simulink model "AUAV3_WITH_SLUGS_SENSOR_AND_CONTROLLER"  (Simulink 8.5)
settings: Solver=FixedStepDiscrete  StartTime=0.0  StopTime=10.0  FixedStep=T  RelTol=1e-3
PreLoadFcn:
  | T = 0.0025;
  | MavlinkBus;
  | 
  | % Baro Altitude Computation
  | % =========================
  | basePressure = 98192.64;
  | baseTemp = 288.215;
  | lapseRate = -0.00198122;
  | baseHeight = 0;
  | 
  | mcuInit
values from neighbouring files (symbols this model uses):
  apSampleTime = 0.01    [mcuInit.m]
  latlong_WP = 1    [mcuInit.m]
  mavlink_gps_raw_int_t = Simulink.Bus    [MavlinkBus.m]    (also in MavlinkBusMarcello.m)
  mavlink_raw_imu_t = Simulink.Bus    [MavlinkBus.m]    (also in MavlinkBusMarcello.m)
  mavlink_scaled_pressure_t = Simulink.Bus    [MavlinkBus.m]    (also in MavlinkBusMarcello.m)
  mavlink_sys_status_t = Simulink.Bus    [MavlinkBus.m]    (also in MavlinkBusMarcello.m)
  Xpoints = [0 0]    [mcuInit.m]
  Ypoints = [0 0]    [mcuInit.m]
  Zpoints = [0 0]    [mcuInit.m]
undefined symbols (not defined in the file or in its folder): A0, A14, A15, A2, A3, A5, A6, accBiasRateLimit, altLatLon, B0, bankCommandLimit, barAdjust, baroCutoff, baroCutTemp, C3, cubeAccelGain16405, cubeGyroGain16405, cubeMagGain16405, D0, D11, D13, D8, daLimit, data, daTrimMax, daTrimMin, deLimit, deTrimMax, deTrimMin, drLimit, drTrimMax, drTrimMin, dtLimit, dtTrimMax, dtTrimMin, F2, F3, G0, G15, gaind, GS_location, gyroBiasRateLimit, IC1max, IPStar, ISA_g, maxAcc, MaxDwnPthStar, maxDynPressure, maxEta, OC1max, P112, P127, P16, P21, P30, P31, P51, P64, P72, P75 ... (+39)
undefined symbols (not defined in the file): baroOffset, baroScale, barTGain1, barTGain2, barTMean1, barTMean2, bda, bde, bdr, bdt, bICda, bICde, bICdr, bICdt, derivativesConstant, lowRateSensorCutoff, mainSensorCutoff, mda, mde, mdr, mdt, mICda, mICde, mICdr, mICdt, pitotOffset, pitotScale, pitTGain1, pitTGain2, pitTMean1, pitTMean2, powerOffset, powerScale, pressureSensorCutoff, tempOffset, tempScale, vzCutoff, xCutoff, yCutoff
libraries: MCHP_Blockset x147, simulink x78, SLUGS_Library x31, aerolibconvert2 x6, aerolibutil x4, aerolibtransform2 x3, dspmtrx3 x2, aerolibobsolete x2
(part 2 of 12)

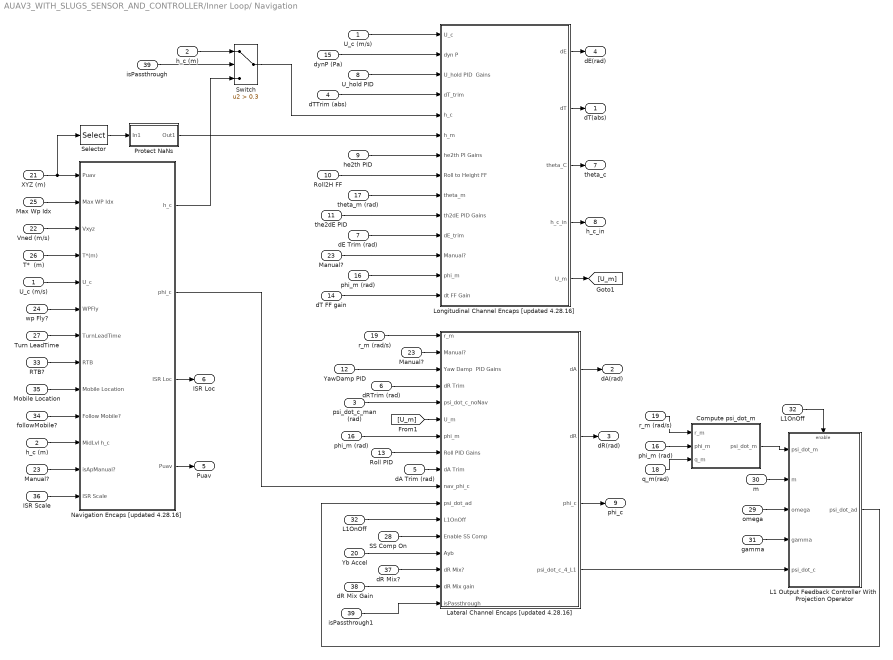
== system AUAV3_WITH_SLUGS_SENSOR_AND_CONTROLLER/Inner Loop/ Navigation ==
  U_c (m/s) : Inport
  h_c (m) : Inport  Port=2
  psi_dot_c_man (rad) : Inport  Port=3
  dTTrim (abs) : Inport  Port=4
  dA Trim (rad) : Inport  Port=5
  dRTrim (rad) : Inport  Port=6
  dE Trim (rad) : Inport  Port=7
  U_hold PID : Inport  Port=8
  he2th PID : Inport  Port=9
  Roll2H FF : Inport  Port=10
  the2dE PID : Inport  Port=11
  YawDamp PID : Inport  Port=12
  "Roll PID " : Inport  Port=13
  dT FF gain : Inport  Port=14
  dynP (Pa) : Inport  Port=15
  phi_m (rad) : Inport  Port=16
  theta_m (rad) : Inport  Port=17
  q_m(rad) : Inport  Port=18
  r_m (rad/s) : Inport  Port=19
  Yb Accel : Inport  Port=20
  XYZ (m) : Inport  Port=21
  Vned (m/s) : Inport  Port=22
  Manual? : Inport  Port=23
  wp Fly? : Inport  Port=24
  Max Wp Idx : Inport  Port=25
  T*  (m) : Inport  Port=26
  Turn LeadTime : Inport  Port=27
  SS Comp On : Inport  Port=28
  omega : Inport  Port=29
  m : Inport  Port=30
  gamma : Inport  Port=31
  L1OnOff : Inport  Port=32
  RTB? : Inport  Port=33
  followMobile? : Inport  Port=34
  Mobile Location : Inport  Port=35
  ISR Scale : Inport  Port=36
  dR Mix? : Inport  Port=37
  dR Mix Gain : Inport  Port=38
  isPassthrough : Inport  Port=39
  Compute psi_dot_m : Subsystem
  L1 Output Feedback Controller With  Projection Operator : Subsystem  TreatAsAtomicUnit=on
  "L1OnOff " : InportShadow  Port=32
  Lateral Channel Encaps [updated 4.28.16] : Subsystem  TreatAsAtomicUnit=on
  Longitudinal Channel Encaps [updated 4.28.16] : Subsystem  TreatAsAtomicUnit=on
  "Manual? " : InportShadow  Port=23
  "Manual?  " : InportShadow  Port=23
  Navigation Encaps [updated 4.28.16] : Subsystem  TreatAsAtomicUnit=on
  Protect NaNs : Subsystem
  Selector : Selector  InputPortWidth=3  Indices=[3]
  Switch : Switch  Criteria=u2 > Threshold  Threshold=0.3  OutDataTypeStr=Inherit: Inherit via back propagation  InputSameDT=on
  "U_c (m/s) " : InportShadow
  "h_c (m) " : InportShadow  Port=2
  isPassthrough1 : InportShadow  Port=39
  "phi_m (rad) " : InportShadow  Port=16
  "phi_m (rad)   " : InportShadow  Port=16
  "r_m (rad/s) " : InportShadow  Port=19
  dT(abs) : Outport
  dA(rad) : Outport  Port=2
  dR(rad) : Outport  Port=3
  dE(rad) : Outport  Port=4
  "Puav " : Outport  Port=5
  ISR Loc : Outport  Port=6
  theta_c : Outport  Port=7
  h_c_in : Outport  Port=8
  phi_c : Outport  Port=9
  wires:
  Manual?/1 -> Longitudinal Channel Encaps [updated 4.28.16]/12(Manual?)
  U_c (m/s)/1 -> Longitudinal Channel Encaps [updated 4.28.16]/1(U_c)
  dynP (Pa)/1 -> Longitudinal Channel Encaps [updated 4.28.16]/2(dyn P)
  Longitudinal Channel Encaps [updated 4.28.16]/1(dE) -> dE(rad)/1
  U_hold PID/1 -> Longitudinal Channel Encaps [updated 4.28.16]/3(U_hold PID  Gains)
  dTTrim (abs)/1 -> Longitudinal Channel Encaps [updated 4.28.16]/4(dT_trim)
  Longitudinal Channel Encaps [updated 4.28.16]/2(dT) -> dT(abs)/1
  Selector/1 -> Protect NaNs/1(In1)
  he2th PID/1 -> Longitudinal Channel Encaps [updated 4.28.16]/7(he2th PI Gains)
  theta_m (rad)/1 -> Longitudinal Channel Encaps [updated 4.28.16]/9(theta_m)
  Longitudinal Channel Encaps [updated 4.28.16]/3(theta_C) -> theta_c/1
  the2dE PID/1 -> Longitudinal Channel Encaps [updated 4.28.16]/10(th2dE PID Gains)
  dE Trim (rad)/1 -> Longitudinal Channel Encaps [updated 4.28.16]/11(dE_trim)
  Longitudinal Channel Encaps [updated 4.28.16]/4(h_c_in) -> h_c_in/1
  r_m (rad/s)/1 -> Lateral Channel Encaps [updated 4.28.16]/1(r_m)
  YawDamp PID/1 -> Lateral Channel Encaps [updated 4.28.16]/3(Yaw Damp  PID Gains)
  dRTrim (rad)/1 -> Lateral Channel Encaps [updated 4.28.16]/4(dR Trim)
  Lateral Channel Encaps [updated 4.28.16]/2(dR) -> dR(rad)/1
  psi_dot_c_man (rad)/1 -> Lateral Channel Encaps [updated 4.28.16]/5(psi_dot_c_noNav)
  phi_m (rad)/1 -> Lateral Channel Encaps [updated 4.28.16]/7(phi_m)
  Lateral Channel Encaps [updated 4.28.16]/3(phi_c) -> phi_c/1
  "Roll PID "/1 -> Lateral Channel Encaps [updated 4.28.16]/8(Roll PID Gains)
  dA Trim (rad)/1 -> Lateral Channel Encaps [updated 4.28.16]/9(dA Trim)
  Longitudinal Channel Encaps [updated 4.28.16]/5(U_m) -> [U_m]
  XYZ (m)/1 -> Selector/1, Navigation Encaps [updated 4.28.16]/1(Puav)
  Max Wp Idx/1 -> Navigation Encaps [updated 4.28.16]/2(Max WP Idx)
  Vned (m/s)/1 -> Navigation Encaps [updated 4.28.16]/3(Vxyz)
  Compute psi_dot_m/1(psi_dot_m) -> L1 Output Feedback Controller With  Projection Operator/1(psi_dot_m)
  m/1 -> L1 Output Feedback Controller With  Projection Operator/2(m)
  omega/1 -> L1 Output Feedback Controller With  Projection Operator/3(omega)
  gamma/1 -> L1 Output Feedback Controller With  Projection Operator/4(gamma)
  "r_m (rad/s) "/1 -> Compute psi_dot_m/1(r_m)
  "phi_m (rad) "/1 -> Compute psi_dot_m/2(phi_m)
  q_m(rad)/1 -> Compute psi_dot_m/3(q_m)
  L1OnOff/1 -> L1 Output Feedback Controller With  Projection Operator/Enable
  L1 Output Feedback Controller With  Projection Operator/1(psi_dot_ad) -> Lateral Channel Encaps [updated 4.28.16]/11(psi_dot_ad)
  "L1OnOff "/1 -> Lateral Channel Encaps [updated 4.28.16]/12(L1OnOff)
  "phi_m (rad)   "/1 -> Longitudinal Channel Encaps [updated 4.28.16]/13(phi_m)
  dT FF gain/1 -> Longitudinal Channel Encaps [updated 4.28.16]/14(dt FF Gain)
  Lateral Channel Encaps [updated 4.28.16]/1(dA) -> dA(rad)/1
  SS Comp On/1 -> Lateral Channel Encaps [updated 4.28.16]/13(Enable SS Comp)
  Yb Accel/1 -> Lateral Channel Encaps [updated 4.28.16]/14(Ayb)
  Lateral Channel Encaps [updated 4.28.16]/4(psi_dot_c_4_L1) -> L1 Output Feedback Controller With  Projection Operator/5(psi_dot_c)
  Protect NaNs/1(Out1) -> Longitudinal Channel Encaps [updated 4.28.16]/6(h_m)
  [U_m] -> Lateral Channel Encaps [updated 4.28.16]/6(U_m)
  "Manual?  "/1 -> Lateral Channel Encaps [updated 4.28.16]/2(Manual?)
  Roll2H FF/1 -> Longitudinal Channel Encaps [updated 4.28.16]/8(Roll to Height FF)
  Navigation Encaps [updated 4.28.16]/2(phi_c) -> Lateral Channel Encaps [updated 4.28.16]/10(nav_phi_c)
  T*  (m)/1 -> Navigation Encaps [updated 4.28.16]/4(T*(m))
  "U_c (m/s) "/1 -> Navigation Encaps [updated 4.28.16]/5(U_c)
  wp Fly?/1 -> Navigation Encaps [updated 4.28.16]/6(WPFly)
  Turn LeadTime/1 -> Navigation Encaps [updated 4.28.16]/7(TurnLeadTime)
  RTB?/1 -> Navigation Encaps [updated 4.28.16]/8(RTB)
  Mobile Location/1 -> Navigation Encaps [updated 4.28.16]/9(Mobile Location)
  followMobile?/1 -> Navigation Encaps [updated 4.28.16]/10(Follow Mobile?)
  "h_c (m) "/1 -> Navigation Encaps [updated 4.28.16]/11(MidLvl h_c)
  "Manual? "/1 -> Navigation Encaps [updated 4.28.16]/12(isApManual?)
  Navigation Encaps [updated 4.28.16]/3(ISR Loc) -> ISR Loc/1
  Navigation Encaps [updated 4.28.16]/4("Puav ") -> "Puav "/1
  dR Mix Gain/1 -> Lateral Channel Encaps [updated 4.28.16]/16(dR Mix gain)
  dR Mix?/1 -> Lateral Channel Encaps [updated 4.28.16]/15(dR Mix?)
  ISR Scale/1 -> Navigation Encaps [updated 4.28.16]/13(ISR Scale)
  isPassthrough/1 -> Switch/2
  h_c (m)/1 -> Switch/1
  Switch/1 -> Longitudinal Channel Encaps [updated 4.28.16]/5(h_c)
  Navigation Encaps [updated 4.28.16]/1(h_c) -> Switch/3
  isPassthrough1/1 -> Lateral Channel Encaps [updated 4.28.16]/17(isPassthrough)

== system AUAV3_WITH_SLUGS_SENSOR_AND_CONTROLLER/MavlinkTX ==
  COMP_ID : Constant  OutDataTypeStr=uint8
  Get Raw IMU : DataStoreRead  DataStoreName=mlRawIMU  DataStoreElements=mlRawIMU
  Get RawGpsInt : DataStoreRead  DataStoreName=mlGpsData
  Get mlAirData : DataStoreRead  DataStoreName=mlAirData  DataStoreElements=mlAirData
  Get mlSysStatus : DataStoreRead  DialogController=Simulink.DDGSource  DataStoreName=mlSysStatus  DataStoreElements=mlSysStatus
  Get time : DataStoreRead  DataStoreName=time_since_boot_usec  DataStoreElements=time_since_boot_usec
  Get time1 : DataStoreRead  DataStoreName=time_since_boot_usec  DataStoreElements=time_since_boot_usec
  Get time2 : DataStoreRead  DataStoreName=time_since_boot_usec  DataStoreElements=time_since_boot_usec
  PackGpsRawInt : MCHP_Blockset/User Functions/C Function Call  ParseFilesChkbx=off  ListFunctions1=Custom Function  Function1=uint16_t PackGpsRawInt(uint8_t system_id, uint8_t component_id, mavlink_gps_raw_int_t mlRawGpsDataInt ,uint32_t time_usec)  AddHeaderDeclaration=on  Function1Type=when block is updated (default)  Fct1BlockIn="system_id  , component_id  , mlRawGpsDataInt  , time_usec"  FctReturnBlockOut=on  DataCollected=0  ORDERING=None  SampleTime=0.2  MCHP_MASTERLINK=|  PinDigitalInput=[]  PinDigitalOutput=[]  PinAnalogInput=[]
      | AUAV3_WITH_SLUGS_SENSOR_AND_CONTROLLER/Microchip Master
      | AUAV V3 Board
      | Busy Flag on D2 (RA6)
  PackHeartBeat : MCHP_Blockset/User Functions/C Function Call  ParseFilesChkbx=off  ListFunctions1=Custom Function  Function1=uint16_t PackHeartBeat(uint8_t system_id, uint8_t component_id)  AddHeaderDeclaration=on  Function1Type=when block is updated (default)  Fct1BlockIn="system_id  , component_id"  FctReturnBlockOut=on  DataCollected=0  ORDERING=None  SampleTime=0.5  MCHP_MASTERLINK=|  PinDigitalInput=[]  PinDigitalOutput=[]  PinAnalogInput=[]
      | AUAV3_WITH_SLUGS_SENSOR_AND_CONTROLLER/Microchip Master
      | AUAV V3 Board
      | Busy Flag on D2 (RA6)
  PackRawIMU : MCHP_Blockset/User Functions/C Function Call  ParseFilesChkbx=off  ListFunctions1=Custom Function  Function1=uint16_t PackRawIMU(uint8_t system_id, uint8_t component_id, mavlink_raw_imu_t mlRawIMUData ,uint32_t time_usec)  AddHeaderDeclaration=on  Function1Type=when block is updated (default)  Fct1BlockIn="system_id  , component_id  , mlRawIMUData  , time_usec"  FctReturnBlockOut=on  DataCollected=0  ORDERING=None  SampleTime=0.02  MCHP_MASTERLINK=|  PinDigitalInput=[]  PinDigitalOutput=[]  PinAnalogInput=[]
      | AUAV3_WITH_SLUGS_SENSOR_AND_CONTROLLER/Microchip Master
      | AUAV V3 Board
      | Busy Flag on D2 (RA6)
  PackScaledPressure : MCHP_Blockset/User Functions/C Function Call  ParseFilesChkbx=off  ListFunctions1=Custom Function  Function1=uint16_t PackScaledPressure(uint8_t system_id, uint8_t component_id, mavlink_scaled_pressure_t mlAirData ,uint32_t time_usec)  AddHeaderDeclaration=on  Function1Type=when block is updated (default)  Fct1BlockIn="system_id  , component_id  , mlAirData  , time_usec"  FctReturnBlockOut=on  DataCollected=0  ORDERING=None  SampleTime=[0.2 0.02]  MCHP_MASTERLINK=|  PinDigitalInput=[]  PinDigitalOutput=[]  PinAnalogInput=[]
      | AUAV3_WITH_SLUGS_SENSOR_AND_CONTROLLER/Microchip Master
      | AUAV V3 Board
      | Busy Flag on D2 (RA6)
  PackSysStatus : MCHP_Blockset/User Functions/C Function Call  ParseFilesChkbx=off  ListFunctions1=Custom Function  Function1=uint16_t PackSysStatus(uint8_t system_id, uint8_t component_id, mavlink_sys_status_t mlSysStatus)  AddHeaderDeclaration=on  Function1Type=when block is updated (default)  Fct1BlockIn="system_id  , component_id  , mlSysStatus"  FctReturnBlockOut=on  DataCollected=0  ORDERING=None  SampleTime=[0.2 0.04]  MCHP_MASTERLINK=|  PinDigitalInput=[]  PinDigitalOutput=[]  PinAnalogInput=[]
      | AUAV3_WITH_SLUGS_SENSOR_AND_CONTROLLER/Microchip Master
      | AUAV V3 Board
      | Busy Flag on D2 (RA6)
  ParamInterfaceResponse : MCHP_Blockset/User Functions/C Function Call  ParseFilesChkbx=off  ListFunctions1=Custom Function  Function1=uint16_t ParameterInterfaceResponse(uint8_t system_id, uint8_t component_id)  AddHeaderDeclaration=on  Function1Type=when block is updated (default)  Fct1BlockIn="system_id  , component_id"  FctReturnBlockOut=on  DataCollected=0  ORDERING=None  SampleTime=[0.2 0.06]  MCHP_MASTERLINK=|  PinDigitalInput=[]  PinDigitalOutput=[]  PinAnalogInput=[]
      | AUAV3_WITH_SLUGS_SENSOR_AND_CONTROLLER/Microchip Master
      | AUAV V3 Board
      | Busy Flag on D2 (RA6)
  ParamInterfaceResponse1 : MCHP_Blockset/User Functions/C Function Call  ParseFilesChkbx=off  ListFunctions1=Custom Function  Function1=uint16_t MissionInterfaceResponse(uint8_t system_id, uint8_t component_id)  AddHeaderDeclaration=on  Function1Type=when block is updated (default)  Fct1BlockIn="system_id  , component_id"  FctReturnBlockOut=on  DataCollected=0  ORDERING=None  SampleTime=[0.2 0.08]  MCHP_MASTERLINK=|  PinDigitalInput=[]  PinDigitalOutput=[]  PinAnalogInput=[]
      | AUAV3_WITH_SLUGS_SENSOR_AND_CONTROLLER/Microchip Master
      | AUAV V3 Board
      | Busy Flag on D2 (RA6)
  SYS_ID : Constant  Value=101  OutDataTypeStr=uint8
  TX_N_Data : MCHP_Blockset/User Functions/C Function Call  ParseFilesChkbx=off  ListFunctions1=Custom Function  Function1=void TxN_Data_OverU1(uint16_t N)  AddHeaderDeclaration=on  Function1Type=when block is updated (default)  Fct1BlockIn=N  FctReturnBlockOut=on  DataCollected=0  ORDERING=None  SampleTime=-1  MCHP_MASTERLINK=|  PinDigitalInput=[]  PinDigitalOutput=[]  PinAnalogInput=[]
      | AUAV3_WITH_SLUGS_SENSOR_AND_CONTROLLER/Microchip Master
      | AUAV V3 Board
      | Busy Flag on D2 (RA6)
  TX_N_Data1 : MCHP_Blockset/User Functions/C Function Call  ParseFilesChkbx=off  ListFunctions1=Custom Function  Function1=void TxN_Data_OverU1(uint16_t N)  AddHeaderDeclaration=on  Function1Type=when block is updated (default)  Fct1BlockIn=N  FctReturnBlockOut=on  DataCollected=0  ORDERING=None  SampleTime=-1  MCHP_MASTERLINK=|  PinDigitalInput=[]  PinDigitalOutput=[]  PinAnalogInput=[]
      | AUAV3_WITH_SLUGS_SENSOR_AND_CONTROLLER/Microchip Master
      | AUAV V3 Board
      | Busy Flag on D2 (RA6)
  TX_N_Data2 : MCHP_Blockset/User Functions/C Function Call  ParseFilesChkbx=off  ListFunctions1=Custom Function  Function1=void TxN_Data_OverU1(uint16_t N)  AddHeaderDeclaration=on  Function1Type=when block is updated (default)  Fct1BlockIn=N  FctReturnBlockOut=on  DataCollected=0  ORDERING=None  SampleTime=-1  MCHP_MASTERLINK=|  PinDigitalInput=[]  PinDigitalOutput=[]  PinAnalogInput=[]
      | AUAV3_WITH_SLUGS_SENSOR_AND_CONTROLLER/Microchip Master
      | AUAV V3 Board
      | Busy Flag on D2 (RA6)
  TX_N_Data3 : MCHP_Blockset/User Functions/C Function Call  ParseFilesChkbx=off  ListFunctions1=Custom Function  Function1=void TxN_Data_OverU1(uint16_t N)  AddHeaderDeclaration=on  Function1Type=when block is updated (default)  Fct1BlockIn=N  FctReturnBlockOut=on  DataCollected=0  ORDERING=None  SampleTime=-1  MCHP_MASTERLINK=|  PinDigitalInput=[]  PinDigitalOutput=[]  PinAnalogInput=[]
      | AUAV3_WITH_SLUGS_SENSOR_AND_CONTROLLER/Microchip Master
      | AUAV V3 Board
      | Busy Flag on D2 (RA6)
  TX_N_Data4 : MCHP_Blockset/User Functions/C Function Call  ParseFilesChkbx=off  ListFunctions1=Custom Function  Function1=void TxN_Data_OverU1(uint16_t N)  AddHeaderDeclaration=on  Function1Type=when block is updated (default)  Fct1BlockIn=N  FctReturnBlockOut=on  DataCollected=0  ORDERING=None  SampleTime=-1  MCHP_MASTERLINK=|  PinDigitalInput=[]  PinDigitalOutput=[]  PinAnalogInput=[]
      | AUAV3_WITH_SLUGS_SENSOR_AND_CONTROLLER/Microchip Master
      | AUAV V3 Board
      | Busy Flag on D2 (RA6)
  TX_N_Data5 : MCHP_Blockset/User Functions/C Function Call  ParseFilesChkbx=off  ListFunctions1=Custom Function  Function1=void TxN_Data_OverU1(uint16_t N)  AddHeaderDeclaration=on  Function1Type=when block is updated (default)  Fct1BlockIn=N  FctReturnBlockOut=on  DataCollected=0  ORDERING=None  SampleTime=-1  MCHP_MASTERLINK=|  PinDigitalInput=[]  PinDigitalOutput=[]  PinAnalogInput=[]
      | AUAV3_WITH_SLUGS_SENSOR_AND_CONTROLLER/Microchip Master
      | AUAV V3 Board
      | Busy Flag on D2 (RA6)
  TX_N_Data6 : MCHP_Blockset/User Functions/C Function Call  ParseFilesChkbx=off  ListFunctions1=Custom Function  Function1=void TxN_Data_OverU1(uint16_t N)  AddHeaderDeclaration=on  Function1Type=when block is updated (default)  Fct1BlockIn=N  FctReturnBlockOut=on  DataCollected=0  ORDERING=None  SampleTime=-1  MCHP_MASTERLINK=|  PinDigitalInput=[]  PinDigitalOutput=[]  PinAnalogInput=[]
      | AUAV3_WITH_SLUGS_SENSOR_AND_CONTROLLER/Microchip Master
      | AUAV V3 Board
      | Busy Flag on D2 (RA6)
  wires:
  Get mlSysStatus/1 -> ?
  PackSysStatus/1 -> TX_N_Data4/1
  Get time2/1 -> ?
  Get mlAirData/1 -> PackScaledPressure/3
  PackScaledPressure/1 -> TX_N_Data3/1
  Get time1/1 -> PackGpsRawInt/4
  Get RawGpsInt/1 -> PackGpsRawInt/3
  PackGpsRawInt/1 -> TX_N_Data2/1
  PackHeartBeat/1 -> TX_N_Data1/1
  PackRawIMU/1 -> TX_N_Data/1
  Get time/1 -> ?
  Get Raw IMU/1 -> PackRawIMU/3
  COMP_ID/1 -> PackRawIMU/2, PackHeartBeat/2, PackGpsRawInt/2, PackScaledPressure/2, PackSysStatus/2, ParamInterfaceResponse1/2, ParamInterfaceResponse/2
  SYS_ID/1 -> PackRawIMU/1, PackHeartBeat/1, PackGpsRawInt/1, PackScaledPressure/1, ParamInterfaceResponse1/1, ParamInterfaceResponse/1, PackSysStatus/1
  ParamInterfaceResponse/1 -> TX_N_Data5/1
  ParamInterfaceResponse1/1 -> TX_N_Data6/1

== system AUAV3_WITH_SLUGS_SENSOR_AND_CONTROLLER/PID Gains [updated 4.28.16] ==
  Constant1 : Constant  Value=PAR_PID_AIRSPEED_P  OutDataTypeStr=uint8
  Constant10 : Constant  Value=PAR_PID_PITCH_FO_P  OutDataTypeStr=uint8
  Constant11 : Constant  Value=PAR_PID_PITCH_FO_I  OutDataTypeStr=uint8
  Constant12 : Constant  Value=PAR_PID_PITC_DT_FF  OutDataTypeStr=uint8
  Constant2 : Constant  Value=PAR_PID_ROLL_CON_P  OutDataTypeStr=uint8
  Constant3 : Constant  Value=PAR_PID_ROLL_CON_D  OutDataTypeStr=uint8
  Constant4 : Constant  Value=PAR_PID_YAW_DAMP_P  OutDataTypeStr=uint8
  Constant5 : Constant  Value=PAR_PID_YAW_DAMP_D  OutDataTypeStr=uint8
  Constant6 : Constant  Value=PAR_PID_HE_TO_PI_P  OutDataTypeStr=uint8
  Constant7 : Constant  Value=PAR_PID_AIRSPEED_D  OutDataTypeStr=uint8
  Constant8 : Constant  Value=PAR_PID_HE_TO_PI_I  OutDataTypeStr=uint8
  Constant9 : Constant  Value=PAR_PID_HEI_ERR_FF  OutDataTypeStr=uint8
  Get Range of Values [navSupport.c] [updated 4.27.16] : MCHP_Blockset/User Functions/C Function Call  ParseFilesChkbx=off  ListFunctions1=Custom Function  Function1=extern void getRangeOfParams(uint8_T u1, uint8_T u2, real32_T* y1);  AddHeaderDeclaration=on  Function1Type=when block is updated (default)  Fct1BlockIn=u1 u2  FctReturnBlockOut=on  Fct1BlockOut=y1[3]  DataCollected=0  ORDERING=None  SampleTime=0.01  MCHP_MASTERLINK=|  PinDigitalInput=[]  PinDigitalOutput=[]  PinAnalogInput=[]
      | AUAV3_WITH_SLUGS_SENSOR_AND_CONTROLLER/Microchip Master
      | AUAV V3 Board
      | Busy Flag on D2 (RA6)
  Get Range of Values [navSupport.c] [updated 4.27.16]1 : MCHP_Blockset/User Functions/C Function Call  ParseFilesChkbx=off  ListFunctions1=Custom Function  Function1=extern void getRangeOfParams(uint8_T u1, uint8_T u2, real32_T* y1);  AddHeaderDeclaration=on  Function1Type=when block is updated (default)  Fct1BlockIn=u1 u2  FctReturnBlockOut=on  Fct1BlockOut=y1[3]  DataCollected=0  ORDERING=None  SampleTime=0.01  MCHP_MASTERLINK=|  PinDigitalInput=[]  PinDigitalOutput=[]  PinAnalogInput=[]
      | AUAV3_WITH_SLUGS_SENSOR_AND_CONTROLLER/Microchip Master
      | AUAV V3 Board
      | Busy Flag on D2 (RA6)
  Get Range of Values [navSupport.c] [updated 4.27.16]2 : MCHP_Blockset/User Functions/C Function Call  ParseFilesChkbx=off  ListFunctions1=Custom Function  Function1=extern void getRangeOfParams(uint8_T u1, uint8_T u2, real32_T* y1);  AddHeaderDeclaration=on  Function1Type=when block is updated (default)  Fct1BlockIn=u1 u2  FctReturnBlockOut=on  Fct1BlockOut=y1[3]  DataCollected=0  ORDERING=None  SampleTime=0.01  MCHP_MASTERLINK=|  PinDigitalInput=[]  PinDigitalOutput=[]  PinAnalogInput=[]
      | AUAV3_WITH_SLUGS_SENSOR_AND_CONTROLLER/Microchip Master
      | AUAV V3 Board
      | Busy Flag on D2 (RA6)
  Get Range of Values [navSupport.c] [updated 4.27.16]3 : MCHP_Blockset/User Functions/C Function Call  ParseFilesChkbx=off  ListFunctions1=Custom Function  Function1=extern void getRangeOfParams(uint8_T u1, uint8_T u2, real32_T* y1);  AddHeaderDeclaration=on  Function1Type=when block is updated (default)  Fct1BlockIn=u1 u2  FctReturnBlockOut=on  Fct1BlockOut=y1[3]  DataCollected=0  ORDERING=None  SampleTime=0.01  MCHP_MASTERLINK=|  PinDigitalInput=[]  PinDigitalOutput=[]  PinAnalogInput=[]
      | AUAV3_WITH_SLUGS_SENSOR_AND_CONTROLLER/Microchip Master
      | AUAV V3 Board
      | Busy Flag on D2 (RA6)
  Get Range of Values [navSupport.c] [updated 4.27.16]4 : MCHP_Blockset/User Functions/C Function Call  ParseFilesChkbx=off  ListFunctions1=Custom Function  Function1=extern void getRangeOfParams(uint8_T u1, uint8_T u2, real32_T* y1);  AddHeaderDeclaration=on  Function1Type=when block is updated (default)  Fct1BlockIn=u1 u2  FctReturnBlockOut=on  Fct1BlockOut=y1[3]  DataCollected=0  ORDERING=None  SampleTime=0.01  MCHP_MASTERLINK=|  PinDigitalInput=[]  PinDigitalOutput=[]  PinAnalogInput=[]
      | AUAV3_WITH_SLUGS_SENSOR_AND_CONTROLLER/Microchip Master
      | AUAV V3 Board
      | Busy Flag on D2 (RA6)
  Get a single Param [navSupport.c] [updated 4.27.16] : MCHP_Blockset/User Functions/C Function Call  ParseFilesChkbx=off  ListFunctions1=Custom Function  Function1=extern real32_T getParamIdx(uint8_T u1);  AddHeaderDeclaration=on  Function1Type=when block is updated (default)  Fct1BlockIn=u1  FctReturnBlockOut=on  Fct1BlockOut=y1  DataCollected=0  ORDERING=None  SampleTime=0.01  MCHP_MASTERLINK=|  PinDigitalInput=[]  PinDigitalOutput=[]  PinAnalogInput=[]
      | AUAV3_WITH_SLUGS_SENSOR_AND_CONTROLLER/Microchip Master
      | AUAV V3 Board
      | Busy Flag on D2 (RA6)
  Get a single Param [navSupport.c] [updated 4.27.16]1 : MCHP_Blockset/User Functions/C Function Call  ParseFilesChkbx=off  ListFunctions1=Custom Function  Function1=extern real32_T getParamIdx(uint8_T u1);  AddHeaderDeclaration=on  Function1Type=when block is updated (default)  Fct1BlockIn=u1  FctReturnBlockOut=on  Fct1BlockOut=y1  DataCollected=0  ORDERING=None  SampleTime=0.01  MCHP_MASTERLINK=|  PinDigitalInput=[]  PinDigitalOutput=[]  PinAnalogInput=[]
      | AUAV3_WITH_SLUGS_SENSOR_AND_CONTROLLER/Microchip Master
      | AUAV V3 Board
      | Busy Flag on D2 (RA6)
  uHold PID : Outport
  he2Th PID : Outport  Port=2
  Roll2H FF : Outport  Port=3
  th2dE PID : Outport  Port=4
  Yaw Damp PID : Outport  Port=5
  Roll PID : Outport  Port=6
  dT FF : Outport  Port=7
  wires:
  Constant7/1 -> Get Range of Values [navSupport.c] [updated 4.27.16]/2
  Constant8/1 -> Get Range of Values [navSupport.c] [updated 4.27.16]1/2
  Constant9/1 -> Get a single Param [navSupport.c] [updated 4.27.16]/1
  Constant3/1 -> Get Range of Values [navSupport.c] [updated 4.27.16]2/2
  Constant5/1 -> Get Range of Values [navSupport.c] [updated 4.27.16]3/2
  Constant11/1 -> Get Range of Values [navSupport.c] [updated 4.27.16]4/2
  Constant12/1 -> Get a single Param [navSupport.c] [updated 4.27.16]1/1
  Constant1/1 -> Get Range of Values [navSupport.c] [updated 4.27.16]/1
  Constant6/1 -> Get Range of Values [navSupport.c] [updated 4.27.16]1/1
  Constant2/1 -> Get Range of Values [navSupport.c] [updated 4.27.16]2/1
  Constant4/1 -> Get Range of Values [navSupport.c] [updated 4.27.16]3/1
  Constant10/1 -> Get Range of Values [navSupport.c] [updated 4.27.16]4/1
  Get Range of Values [navSupport.c] [updated 4.27.16]/1 -> uHold PID/1
  Get Range of Values [navSupport.c] [updated 4.27.16]1/1 -> he2Th PID/1
  Get a single Param [navSupport.c] [updated 4.27.16]/1 -> Roll2H FF/1
  Get Range of Values [navSupport.c] [updated 4.27.16]2/1 -> Roll PID/1
  Get Range of Values [navSupport.c] [updated 4.27.16]3/1 -> Yaw Damp PID/1
  Get Range of Values [navSupport.c] [updated 4.27.16]4/1 -> th2dE PID/1
  Get a single Param [navSupport.c] [updated 4.27.16]1/1 -> dT FF/1

== system AUAV3_WITH_SLUGS_SENSOR_AND_CONTROLLER/Pilot LED and HIL Control Pins ==
  In1 : Inport
  HIL_Status : Inport  Port=2
  Data Type Conversion1 : DataTypeConversion  OutDataTypeStr=boolean
  Data Type Conversion2 : DataTypeConversion  OutDataTypeStr=boolean
  HIL Attitude On/Off Switch : MCHP_Blockset/Digital IO/Digital Output  PORT=Dynamic Options  PORT_TXT="B   [ 0 : 15 ]"  PIN=6  PACK=off  SIMULTANEOUS=off  READPREVIOUS=off  ORDERING=None  SampleTime=-1  MCHP_MASTERLINK=|
      | AUAV3_WITH_SLUGS_SENSOR_AND_CONTROLLER/Microchip Master
      | AUAV V3 Board
      | Busy Flag on D2 (RA6)
  HIL On/Off Switch : MCHP_Blockset/Digital IO/Digital Output  PORT=Dynamic Options  PORT_TXT="E   [ 0 : 9 ]"  PIN=9  PACK=off  SIMULTANEOUS=off  READPREVIOUS=off  ORDERING=None  SampleTime=-1  MCHP_MASTERLINK=|
      | AUAV3_WITH_SLUGS_SENSOR_AND_CONTROLLER/Microchip Master
      | AUAV V3 Board
      | Busy Flag on D2 (RA6)
  Off : Constant  Value=0  OutDataTypeStr=boolean
  Terminator : Terminator
  VI Sensor D01 : MCHP_Blockset/Digital IO/Digital Output  PORT=Dynamic Options  PORT_TXT="G   [ 0  1  2  3  6  7  8  9  12  13  14  15 ]"  PIN=8  PACK=off  SIMULTANEOUS=off  READPREVIOUS=off  ORDERING=None  SampleTime=-1  MCHP_MASTERLINK=|
      | AUAV3_WITH_SLUGS_SENSOR_AND_CONTROLLER/Microchip Master
      | AUAV V3 Board
      | Busy Flag on D2 (RA6)
  VI Sensor D02 : MCHP_Blockset/Digital IO/Digital Output  PORT=Dynamic Options  PORT_TXT="G   [ 0  1  2  3  6  7  8  9  12  13  14  15 ]"  PIN=9  PACK=off  SIMULTANEOUS=off  READPREVIOUS=off  ORDERING=None  SampleTime=-1  MCHP_MASTERLINK=|
      | AUAV3_WITH_SLUGS_SENSOR_AND_CONTROLLER/Microchip Master
      | AUAV V3 Board
      | Busy Flag on D2 (RA6)
  wires:
  HIL_Status/1 -> Data Type Conversion1/1
  Data Type Conversion1/1 -> HIL On/Off Switch/1, HIL Attitude On/Off Switch/1
  In1/1 -> Data Type Conversion2/1
  Data Type Conversion2/1 -> Terminator/1
  Off/1 -> VI Sensor D01/1, VI Sensor D02/1

== system AUAV3_WITH_SLUGS_SENSOR_AND_CONTROLLER/Position and Attitude Filter [updated 5.13.16] ==
  A_sens(m/s^2) : Inport
  Omega (rad/s) : Inport  Port=2
  GPSMain : Inport  Port=3
  Baro Alt (m) : Inport  Port=4
  "A_sens(m/s^2) " : InportShadow
  Attitude Complimentary Filter COG : Subsystem
  COG.SOG2V : Subsystem
  Checks if FixType is 3 [updateSensorMCUState.c]1 : MCHP_Blockset/User Functions/C Function Call  ParseFilesChkbx=off  ListFunctions1=Custom Function  Function1=uint8_T isFixValid();  AddHeaderDeclaration=on  Function1Type=when block is updated (default)  FctReturnBlockOut=on  DataCollected=0  ORDERING=None  SampleTime=.01  MCHP_MASTERLINK=|  PinDigitalInput=[]  PinDigitalOutput=[]  PinAnalogInput=[]
      | AUAV3_WITH_SLUGS_SENSOR_AND_CONTROLLER/Microchip Master
      | AUAV V3 Board
      | Busy Flag on D2 (RA6)
  Compute GS Location : Subsystem
  Demux : Demux  Outputs=5
  Enabled Subsystem : Subsystem  TreatAsAtomicUnit=on
  GPS Update : Subsystem  mask{T=0.01}
      mask prompts: T "Sample Time"
  Geod2LTP1 : Subsystem
      mask help:
      | This block provides transformation of the Geodetic coordinates
      | to the LTP coorinate system. The block uses two consecutive transformations
      | (Geodetic -> ECEF ->LTP).
      | Geodetic coordinates of the LTP origin should also be predetermined.
      mask Help: Oops!
      mask Display: plot(0,0,100,100,[45,40,35,40,40],[85,95,85,95,40],[85,95,85,95,40],[35,40,45,40,40],[60,40,10,20,10,14],[70,40,10,13,10,20],[56,45],[70,70],[60,60],[50,60],[60,60],[30,40],[50,60],[20,20],[30,40],[20,20],[45,55],[35,25],[75,65],[35,25])
  Get the GS Location [updateSensorMCUState.c] : MCHP_Blockset/User Functions/C Function Call  ParseFilesChkbx=off  ListFunctions1=Custom Function  Function1=void getGSLocation(real32_T* y1);  AddHeaderDeclaration=on  Function1Type=when block is updated (default)  FctReturnBlockOut=on  Fct1BlockOut=y1[3]  DataCollected=0  ORDERING=None  SampleTime=.01  MCHP_MASTERLINK=|  PinDigitalInput=[]  PinDigitalOutput=[]  PinAnalogInput=[]
      | AUAV3_WITH_SLUGS_SENSOR_AND_CONTROLLER/Microchip Master
      | AUAV V3 Board
      | Busy Flag on D2 (RA6)
  Position Filter [updated 5.13.16] : Subsystem
  "[1 1 -1]" : Gain  Gain=[1 1 -1]
  get Height : Selector  InputPortWidth=3  Indices=[1]
  euler_hat (rad) : Outport
  pqr_hat (rad/s) : Outport  Port=2
  Pxyz_hat (m) : Outport  Port=3
  Vned_hat (m/s) : Outport  Port=4
  GyroBias (rad/s) : Outport  Port=5
  Accel Bias (m/s) : Outport  Port=6
  wires:
  Position Filter [updated 5.13.16]/1(Vxyd_hat) -> Vned_hat (m/s)/1, Attitude Complimentary Filter COG/4(Vxyd_hat)
  Position Filter [updated 5.13.16]/2(Pxyd_hat) -> Pxyz_hat (m)/1
  Position Filter [updated 5.13.16]/3(acc_bias) -> Attitude Complimentary Filter COG/5(acc_bias), Accel Bias (m/s)/1
  Attitude Complimentary Filter COG/1(euler_hat) -> euler_hat (rad)/1
  Attitude Complimentary Filter COG/2(pqr_hat) -> pqr_hat (rad/s)/1
  Attitude Complimentary Filter COG/3(Gyro Bias) -> GyroBias (rad/s)/1
  GPSMain/1 -> Demux/1
  Demux/1 -> Geod2LTP1/3("Lat, deg(GPS)")
  Demux/2 -> Geod2LTP1/4("Lon, deg(GPS)")
  Demux/3 -> Geod2LTP1/5(Hight,m(GPS))
  Compute GS Location/2(R_in) -> Geod2LTP1/2(GS ECEF)
  Compute GS Location/1("Lat, Lon") -> Geod2LTP1/1(GS Lat,Lon)
  GPS Update/1(Update?) -> Position Filter [updated 5.13.16]/1(NewGPS)
  A_sens(m/s^2)/1 -> Attitude Complimentary Filter COG/1(A_sens)
  Omega (rad/s)/1 -> Attitude Complimentary Filter COG/3(Gyros)
  "[1 1 -1]"/1 -> Position Filter [updated 5.13.16]/4(GPS_XYD)
  [XY_Orient] -> Attitude Complimentary Filter COG/2(XY Orient)
  Baro Alt (m)/1 -> Position Filter [updated 5.13.16]/2(Baro Alt)
  COG.SOG2V/1(Vnorth) -> Position Filter [updated 5.13.16]/5(Vnorth)
  COG.SOG2V/2(Veast) -> Position Filter [updated 5.13.16]/6(Veast)
  COG.SOG2V/3(XY Orient) -> [XY_Orient]
  Attitude Complimentary Filter COG/4(RL2B) -> [RL2B]
  [RL2B] -> Position Filter [updated 5.13.16]/3(RLT2B)
  Enabled Subsystem/1(Out1) -> GPS Update/1(XYZ), "[1 1 -1]"/1
  Geod2LTP1/1("NEU, m") -> Enabled Subsystem/1(In1)
  Demux/4 -> Enabled Subsystem/2(In2)
  Demux/5 -> Enabled Subsystem/3(In3)
  Enabled Subsystem/2(Out2) -> COG.SOG2V/1(COG_D)
  Enabled Subsystem/3(Out3) -> COG.SOG2V/2(SOG), Position Filter [updated 5.13.16]/7(SOG)
  "A_sens(m/s^2) "/1 -> Position Filter [updated 5.13.16]/8(A_sens(m/s^2))
  get Height/1 -> Position Filter [updated 5.13.16]/9(Base Height (m))
  Get the GS Location [updateSensorMCUState.c]/1 -> Compute GS Location/1(GS Location), get Height/1
  Checks if FixType is 3 [updateSensorMCUState.c]1/1 -> Enabled Subsystem/Enable

== system AUAV3_WITH_SLUGS_SENSOR_AND_CONTROLLER/Read Barometer BMP180 ==
  BMP 180 Temperature Compensation See datasheet : Subsystem
  "BUS I2C Initialize BMP180 Read P, Convert T° @100Hz" : MCHP_Blockset/BUS I2C/BUS I2C MASTER  I2CRef=2  I2C_IntPriority=6  I2Csequence_txt="Initial-Configuration$     ---     $Start$Write Address:{[0x77]}    % BMP180 Address$Write Data (x1)  Write:{[0xF6]}  $Re-Start    % Re-Start when not followed with either Read or Write action rethrow Address$Read Data (x2)  Read:{adc out}    % Read converted value$Stop$Start$Write Address:{[0x77]}    % BMP180 Address$Write Data (x1)  Write:{[0xF4 0x2E]}      % Start T° Conversion$Stop"  I2Csequence_num=[BFF0000000000000 40E0600000000000 41186A0000000000 4118666E3C87173F]$[4070000000000000]$[3FF0000000000000 40E0200000000000 40F86A0000000000 40F866E066594CA2]$[4040000000000000 0000000000000000 0000000000000000 405DC00000000000]$[4050000000000000 3FF0000000000000 0000000000000000 406EC00000000000]$[4008000000000000 40E0000000000000 40F86A0000000000 410065D9C7810E65]$[4060000000000000 4000000000000000]$[4000000000000000 40E0000000000000 40F86A0000000000 410065D9C7810E65]$[3FF0000000000000 40E0000000000000 40F86A0000000000 410065D9C7810E65]$[4040000000000000 0000000000000000 0000000000000000 405DC00000000000]$[4050000000000000 3FF0000000000000 0000000000000000 406E800000000000 4047000000000000]$[4000000000000000 40E0000000000000 40F86A0000000000 410065D9C7810E65]  InitialConfigurationNum=0  PIN_SDA_TXT=A3 / Pin[59]  PIN_SCL_TXT=A2 / Pin[58]  S_INPUT="[5  5]"  S_OUTPUT=[5]  S_INPUT_Size="[2  2]"  S_OUTPUT_Size=[4]  BlockingMode=off  SampleTime=[ .01]  MCHP_MASTERLINK=|  MCHP_PORT={I2C 2 Clock}{SCL2}13:0:A2;{I2C 2 SDA}{SDA2}13:0:A3;  ORDERING=0
      | AUAV3_WITH_SLUGS_SENSOR_AND_CONTROLLER/Microchip Master
      | AUAV V3 Board
      | Busy Flag on D2 (RA6)
  "BUS I2C Initialize BMP180 Read T°, Convert P @ 100Hz" : MCHP_Blockset/BUS I2C/BUS I2C MASTER  I2CRef=2  I2C_IntPriority=6  I2Csequence_txt="Initial-Configuration$     ---     $Start$Write Address:{[0x77]}    % BMP180 Address$Write Data (x1)  Write:{[0xF6]}  $Re-Start    % Re-Start when not followed with either Read or Write action rethrow Address$Read Data (x2)  Read:{adc out}    % Read converted value$Stop$Start$Write Address:{[0x77]}    % BMP180 Address$Write Data (x1)  Write:{[0xF4 0x34]}      % Start T° Conversion$Stop"  I2Csequence_num=[BFF0000000000000 40E0600000000000 41186A0000000000 4118666E3C87173F]$[4070000000000000]$[3FF0000000000000 40E0200000000000 40F86A0000000000 40F866E066594CA2]$[4040000000000000 0000000000000000 0000000000000000 405DC00000000000]$[4050000000000000 3FF0000000000000 0000000000000000 406EC00000000000]$[4008000000000000 40E0000000000000 40F86A0000000000 410065D9C7810E65]$[4060000000000000 4000000000000000]$[4000000000000000 40E0000000000000 40F86A0000000000 410065D9C7810E65]$[3FF0000000000000 40E0000000000000 40F86A0000000000 410065D9C7810E65]$[4040000000000000 0000000000000000 0000000000000000 405DC00000000000]$[4050000000000000 3FF0000000000000 0000000000000000 406E800000000000 404A000000000000]$[4000000000000000 40E0000000000000 40F86A0000000000 410065D9C7810E65]  InitialConfigurationNum=0  PIN_SDA_TXT=A3 / Pin[59]  PIN_SCL_TXT=A2 / Pin[58]  S_INPUT="[5  5]"  S_OUTPUT=[5]  S_INPUT_Size="[2  2]"  S_OUTPUT_Size=[4]  BlockingMode=off  SampleTime=[.01]  MCHP_MASTERLINK=|  MCHP_PORT={I2C 2 Clock}{SCL2}13:0:A2;{I2C 2 SDA}{SDA2}13:0:A3;  ORDERING=0
      | AUAV3_WITH_SLUGS_SENSOR_AND_CONTROLLER/Microchip Master
      | AUAV V3 Board
      | Busy Flag on D2 (RA6)
  Baro Altimeter : Subsystem  AncestorBlock=SLUGS_Library/Sensor Blocks/Baro Alt/Baro Altimeter
  Constant : Constant  Value=0  OutDataTypeStr=uint16
  Data Type Conversion10 : DataTypeConversion  OutDataTypeStr=int16
  Data Type Conversion7 : DataTypeConversion  OutDataTypeStr=int16
  Data Type Conversion8 : DataTypeConversion  OutDataTypeStr=int16
  Data Type Conversion9 : DataTypeConversion  OutDataTypeStr=single
  Delay : Delay  DelayLength=1  InitialCondition=1  InputProcessing=Inherited  SampleTime=.01
  Demux4 : Demux  Outputs=2
  Demux5 : Demux  Outputs=2
  Gain21 : Gain  Gain=10  OutDataTypeStr=int16
  I2C Initialisation Read EEPROM Calibration data Once (Blocking Function) : Subsystem
  LPF 1Hz : Subsystem  Tag=FilterWizardSubSystem
      settings: ErrorFcn=dspFilterRealizedInBasicElemsAlgLoopErrFcnCallback
  LPF 1Hz1 : Subsystem  Tag=FilterWizardSubSystem
      settings: ErrorFcn=dspFilterRealizedInBasicElemsAlgLoopErrFcnCallback
  Pack : Subsystem
  Pack1 : Subsystem
  Rate Transition1 : RateTransition  Deterministic=off  OutPortSampleTime=.01
  Script Pressure to Altitude : simulink/Model-Wide Utilities/DocBlock  DocumentType=Text
      content=|
      | %% The script to compute the lookup table to translate pressure from Pascal unit (Pa) to meters (m) here after
      |
      | func = '44331.5-4946.62*x.^0.190263';   % Model from Pressure (Pa) to altitude (m)
      |
      | xmin = 35000;  xmax = 101325; % Min and max pressure
      | xdt = ufix(32); xscale = 1; % x scaling
      |
      | ydt = ufix(16);
      | yscale = 2^-3;  % y output is altitude, in m. Max value is 8000 thus 13 bits are required for integer part and 3 can be used as fractional part.
      | % y LSB is 12.5 cm
      |
      | rndmeth = 'Floor';
      | errmax = [.2];
      | nptsmax = 256;
      | %spacing = 'even';
      |
      | % Compute lookup table (might take few seconds to compute)
      | [xdata,ydata,errworst] = fixpt_look1_func_approx(func,xmin,xmax,xdt,xscale,ydt,yscale,rndmeth,errmax,nptsmax);
      | % Check results
      | fixpt_look1_func_plot(xdata,ydata,func,xmin,xmax,xdt,xscale,ydt,yscale,rndmeth);
  Update RawPressure : DataStoreWrite  DataStoreName=mlRawPressureData  DataStoreElements=mlRawPressureData.press_abs#mlRawPressureData.temperature
  Update ScaledPressure : DataStoreWrite  DataStoreName=mlAirData  DataStoreElements=mlAirData.temperature#mlAirData.press_abs
  wires:
  "BUS I2C Initialize BMP180 Read T°, Convert P @ 100Hz"/1 -> Demux4/1
  "BUS I2C Initialize BMP180 Read P, Convert T° @100Hz"/1 -> Demux5/1
  Demux4/1 -> Pack/1(Hi)
  Demux4/2 -> Pack/2(Low)
  Demux5/1 -> Pack1/1(Hi)
  Demux5/2 -> Pack1/2(Low)
  Pack1/1(Out1) -> LPF 1Hz1/1(Input)  "UP"
  Pack/1(Out1) -> LPF 1Hz/1(Input)  "UT"
  LPF 1Hz/1(Output) -> Data Type Conversion7/1, BMP 180 Temperature Compensation See datasheet/12(UT)  "U3 CH3"
  LPF 1Hz1/1(Output) -> Rate Transition1/1
  BMP 180 Temperature Compensation See datasheet/2(p) -> Baro Altimeter/1(Static (Pa))  "Pressute (Pa)"
  Constant/1 -> Delay/1
  I2C Initialisation Read EEPROM Calibration data Once (Blocking Function)/1(Out1) -> BMP 180 Temperature Compensation See datasheet/1(AC1)
  I2C Initialisation Read EEPROM Calibration data Once (Blocking Function)/2(Out2) -> BMP 180 Temperature Compensation See datasheet/2(AC2)
  I2C Initialisation Read EEPROM Calibration data Once (Blocking Function)/3(Out3) -> BMP 180 Temperature Compensation See datasheet/3(AC3)
  I2C Initialisation Read EEPROM Calibration data Once (Blocking Function)/4(Out4) -> BMP 180 Temperature Compensation See datasheet/4(AC4)
  I2C Initialisation Read EEPROM Calibration data Once (Blocking Function)/5(Out5) -> BMP 180 Temperature Compensation See datasheet/5(AC5)
  I2C Initialisation Read EEPROM Calibration data Once (Blocking Function)/6(Out6) -> BMP 180 Temperature Compensation See datasheet/6(AC6)
  I2C Initialisation Read EEPROM Calibration data Once (Blocking Function)/7(Out7) -> BMP 180 Temperature Compensation See datasheet/7(B1)
  I2C Initialisation Read EEPROM Calibration data Once (Blocking Function)/8(Out8) -> BMP 180 Temperature Compensation See datasheet/8(B2)
  I2C Initialisation Read EEPROM Calibration data Once (Blocking Function)/9(Out9) -> BMP 180 Temperature Compensation See datasheet/9(MB)
  I2C Initialisation Read EEPROM Calibration data Once (Blocking Function)/10(Out10) -> BMP 180 Temperature Compensation See datasheet/10(MC)
  I2C Initialisation Read EEPROM Calibration data Once (Blocking Function)/11(Out11) -> BMP 180 Temperature Compensation See datasheet/11(MD)
  Delay/1 -> I2C Initialisation Read EEPROM Calibration data Once (Blocking Function)/Enable
  Rate Transition1/1 -> Data Type Conversion8/1, BMP 180 Temperature Compensation See datasheet/13(UP)  "U3 CH4"
  Data Type Conversion7/1 -> Update RawPressure/1
  Data Type Conversion8/1 -> Update RawPressure/2
  BMP 180 Temperature Compensation See datasheet/1(T) -> Gain21/1  "Temp (deg) * 10"
  Baro Altimeter/1(Altitude) -> Data Type Conversion9/1  "U3 CH3"
  Data Type Conversion10/1 -> Update ScaledPressure/1
  Gain21/1 -> Data Type Conversion10/1
  Data Type Conversion9/1 -> Update ScaledPressure/2

== system AUAV3_WITH_SLUGS_SENSOR_AND_CONTROLLER/Read MPU600 and HMC5883 ==
  BUS I2C Read HMC5883 Magn (50 Hz) : MCHP_Blockset/BUS I2C/BUS I2C MASTER  I2CRef=2  I2C_IntPriority=6  I2Csequence_txt="Initial-Configuration$     ---     $Start$Write Address:{[0x1E]}    % HMC5883L Address$Write Data (x1)  Write:{[0x3]}  $Stop$Start$Write Address:{[0x1E]}    % HMC5883L Address$Read Data (x6)  Read:{Out 5}$Stop"  I2Csequence_num=[BFF0000000000000 40E0600000000000 41186A0000000000 4118666E3C87173F]$[4070000000000000]$[3FF0000000000000 40E0200000000000 40F86A0000000000 40F866E066594CA2]$[4040000000000000 0000000000000000 0000000000000000 403E000000000000]$[4050000000000000 3FF0000000000000 0000000000000000 4008000000000000]$[4000000000000000 40E0600000000000 40F86A0000000000 40F866E066594CA2]$[3FF0000000000000 40E0200000000000 40F86A0000000000 40F866E066594CA2]$[4040000000000000 0000000000000000 0000000000000000 403E000000000000]$[4060000000000000 4018000000000000]$[4000000000000000 40E0600000000000 40F86A0000000000 40F866E066594CA2]  InitialConfigurationNum=0  PIN_SDA_TXT=A3 / Pin[59]  PIN_SCL_TXT=A2 / Pin[58]  S_INPUT="[5  5]"  S_OUTPUT=[5]  S_INPUT_Size="[2  2]"  S_OUTPUT_Size=[4]  BlockingMode=off  SampleTime=0.01  MCHP_MASTERLINK=|  MCHP_PORT={I2C 2 Clock}{SCL2}13:0:A2;{I2C 2 SDA}{SDA2}13:0:A3;  ORDERING=0
      | AUAV3_WITH_SLUGS_SENSOR_AND_CONTROLLER/Microchip Master
      | AUAV V3 Board
      | Busy Flag on D2 (RA6)
  "BUS SPI Read MPU 6050 Axyz, T°, Gxyz (1 kHz)" : MCHP_Blockset/BUS SPI/BUS SPI  SPIRef=1  DMA="[0  2  3]"  SPI_IntPriority=5  SPIsequence_txt="Initial-Configuration$     ---     $Set Port E4 / Pin[100] to 0    % /CS$Write only (x1)  Write:{[0xBA00]}      % read one byte before$Read only (x3)  Read:{Axyz}    % Accelerometers$Read only (x1)  Read:{T°}    % Temperature$Read only (x3)  Read:{Gxyz}    % rate gyros$Set Port E4 / Pin[100] to 1    % /CS"  SPIsequence_num=[BFF0000000000000 4091D00000000000 0000000000000000 40E0000000000000 4116409C00000000 4116409D55555555]$[4070000000000000]$[4010000000000000 4051000000000000 0000000000000000]$[3FF0000000000000 3FF0000000000000 0000000000000000 40E7400000000000]$[4000000000000000 4008000000000000]$[4000000000000000 3FF0000000000000]$[4000000000000000 4008000000000000]$[4010000000000000 4051000000000000 3FF0000000000000]  PIN_SDI_TXT=E3 / P83 / Pin[99]  PIN_SDO_TXT=E2 / P82 / Pin[98]  PIN_SCK_TXT=G15 / P127 / Pin[1]  PIN_SS_TXT=B0 / Pin[21]  S_INPUT="[5  5]"  S_OUTPUT=[5]  S_INPUT_Size="[2  2]"  S_OUTPUT_Size=[4]  BlockingMode=off  SampleTime=[.01]  MCHP_MASTERLINK=|  MCHP_PORT={SPI 1 input}{SDI1}12:0:P83;{SPI 1 output}{SDO1}12:1:P82;{SPI 1 Clock output}{SCK1}12:1:P127;{SPI 1 Digital output}{SPI1-DOU}12:1:E4;{SPI 1 Digital output}{SPI1-DOU}12:1:E4;  ORDERING=0
      | AUAV3_WITH_SLUGS_SENSOR_AND_CONTROLLER/Microchip Master
      | AUAV V3 Board
      | Busy Flag on D2 (RA6)
  Data Type Conversion{,1..5} (6 alike) : DataTypeConversion  OutDataTypeStr=int16
  Demux1 : Demux  Outputs=3
  Demux2 : Demux  Outputs=3
  Demux3 : Demux  Outputs=6
  Subsystem10 : Subsystem
  Subsystem8 : Subsystem
  Subsystem9 : Subsystem
  Update MPU_T : DataStoreWrite  DataStoreName=MPU_T  DataStoreElements=MPU_T
  Update Raw IMU DATA : DataStoreWrite  DataStoreName=mlRawIMU  DataStoreElements=mlRawIMU.xacc#mlRawIMU.yacc#mlRawIMU.zacc#mlRawIMU.xgyro#mlRawIMU.ygyro#mlRawIMU.zgyro#mlRawIMU.xmag#mlRawIMU.ymag#mlRawIMU.zmag
  wires:
  "BUS SPI Read MPU 6050 Axyz, T°, Gxyz (1 kHz)"/1 -> Demux1/1  "U1 CH8"
  "BUS SPI Read MPU 6050 Axyz, T°, Gxyz (1 kHz)"/3 -> Demux2/1
  Demux1/3 -> Data Type Conversion2/1  "U1 CH3"
  Demux1/1 -> Data Type Conversion/1  "U1 CH1"
  Demux1/2 -> Data Type Conversion1/1  "U1 CH2"
  Demux2/1 -> Data Type Conversion3/1  "U1 CH5"
  Demux2/2 -> Data Type Conversion4/1  "U1 CH6"
  Demux2/3 -> Data Type Conversion5/1  "U1 CH7"
  BUS I2C Read HMC5883 Magn (50 Hz)/1 -> Demux3/1
  Demux3/1 -> Subsystem8/1(Hi)
  Demux3/2 -> Subsystem8/2(Low)
  Demux3/3 -> Subsystem9/1(Hi)
  Demux3/4 -> Subsystem9/2(Low)
  Demux3/6 -> Subsystem10/2(Low)
  Demux3/5 -> Subsystem10/1(Hi)
  Subsystem9/1(Out1) -> Update Raw IMU DATA/8  "U1 CH9"
  Subsystem8/1(Out1) -> Update Raw IMU DATA/7  "U1 CH8"
  Subsystem10/1(Out1) -> Update Raw IMU DATA/9  "U1 CH10"
  Data Type Conversion/1 -> Update Raw IMU DATA/1
  Data Type Conversion1/1 -> Update Raw IMU DATA/2
  Data Type Conversion2/1 -> Update Raw IMU DATA/3
  Data Type Conversion3/1 -> Update Raw IMU DATA/4
  Data Type Conversion4/1 -> Update Raw IMU DATA/5
  Data Type Conversion5/1 -> Update Raw IMU DATA/6
  "BUS SPI Read MPU 6050 Axyz, T°, Gxyz (1 kHz)"/2 -> Update MPU_T/1  "U1 CH4"

== system AUAV3_WITH_SLUGS_SENSOR_AND_CONTROLLER/Sensor Data [updated 4.28.16] ==
  Data Type Conversion : DataTypeConversion  OutDataTypeStr=uint8  SampleTime=0.01
  Enable HIL from  Control MCU1 : MCHP_Blockset/Digital IO/Digital Input  PORT=Dynamic Options  PORT_TXT="D   [ 0 : 15 ]"  PIN=[2]  PACK=off  SIMULTANEOUS=off  ORDERING=None  SampleTime=.01  MCHP_PORT={Digital In}{DIN}2:0:D2;  MCHP_MASTERLINK=|
      | AUAV3_WITH_SLUGS_SENSOR_AND_CONTROLLER/Microchip Master
      | AUAV V3 Board
      | Busy Flag on D2 (RA6)
  Raw HIL  Readings : Subsystem
  Sensor Suite : Subsystem
  Omega (rad/s) : Outport
  Accel (m/s^2) : Outport  Port=2
  Mag (mG) : Outport  Port=3
  Baro Alt (m) : Outport  Port=4
  HIL On? : Outport  Port=5
  GPS : Outport  Port=6
  wires:
  Raw HIL  Readings/1(Raw Msg) -> Sensor Suite/2(Raw HIL)
  Enable HIL from  Control MCU1/1 -> Raw HIL  Readings/Enable, Sensor Suite/1(D2), Data Type Conversion/1
  Data Type Conversion/1 -> HIL On?/1
  Sensor Suite/1(Omega (rad/s)) -> Omega (rad/s)/1
  Sensor Suite/2(Accel (m/s^2)) -> Accel (m/s^2)/1
  Sensor Suite/3(Mag (mG)) -> Mag (mG)/1
  Sensor Suite/4(Baro Alt (m)) -> Baro Alt (m)/1
  Sensor Suite/5(GPS) -> GPS/1
